simulink model "sim_v1_PD_single_coil"  (R2021b)
settings: Solver=VariableStepAuto  StartTime=0.0  StopTime=10.0  RelTol=1e-3
undefined symbols (not defined in the file or in its folder): kv, L, m, R
libraries: slpidlib x1
settings Model: Creator=User  LastModifiedBy=User

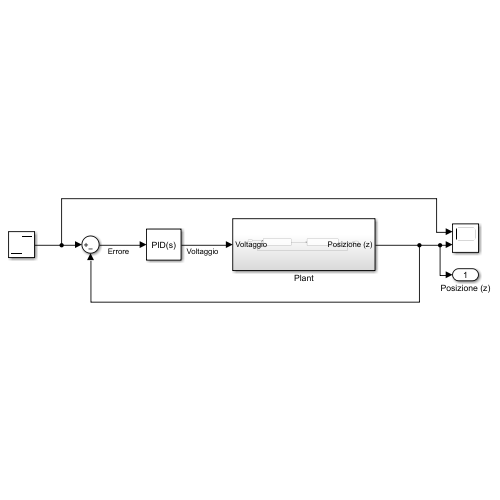
[thumbnail: Simulink's stored preview of the top-level diagram]
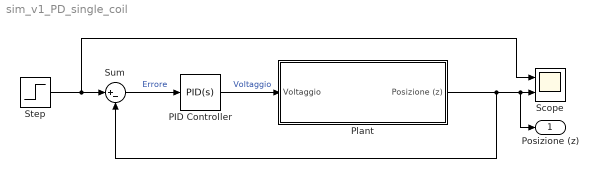
== system sim_v1_PD_single_coil ==
  PID Controller : slpidlib/PID Controller  Controller=PID  Form=Parallel  TimeDomain=Continuous-time  UseExternalTs=off  SampleTime=-1  IntegratorMethod=Forward Euler  FilterMethod=Forward Euler  ControllerParametersSource=internal  P=-1  I=1  D=1  UseFilter=on  N=100  TunerSelectOption=Transfer Function Based (PID Tuner App)  InitialConditionSource=internal  InitialConditionForIntegrator=0  InitialConditionForFilter=0  DifferentiatorICPrevScaledInput=0  ExternalReset=none  TrackingMode=off  Kt=1  LimitOutput=off  SatLimitsSource=internal  UpperSaturationLimit=inf  LowerSaturationLimit=-inf  LinearizeAsGain=on  AntiWindupMode=none  Kb=1  POutMin=[]  POutMax=[]  IOutMin=[]  IOutMax=[]  DOutMin=[]  DOutMax=[]  NOutMin=[]  NOutMax=[]  SumOutMin=[]  SumOutMax=[]  SaturationOutMin=[]  SaturationOutMax=[]  PParamMin=[]  PParamMax=[]  IParamMin=[]  IParamMax=[]  DParamMin=[]  DParamMax=[]  NParamMin=[]  NParamMax=[]  KbParamMin=[]  KbParamMax=[]  KtParamMin=[]  KtParamMax=[]  KbOutMin=[]  KbOutMax=[]  KtOutMin=[]  KtOutMax=[]  IntegratorOutMin=[]  IntegratorOutMax=[]  FilterOutMin=[]  FilterOutMax=[]  SumI1OutMin=[]  SumI1OutMax=[]  SumI2OutMin=[]  SumI2OutMax=[]  SumI3OutMin=[]  SumI3OutMax=[]  SumI4OutMin=[]  SumI4OutMax=[]  SumDOutMin=[]  SumDOutMax=[]  DifferentiatorOutMin=[]  DifferentiatorOutMax=[]  FilterDiffOutCoefMin=[]  FilterDiffOutCoefMax=[]  ReciprocalOutMin=[]  ReciprocalOutMax=[]  SumDenOutMin=[]  SumDenOutMax=[]  SumNumOutMin=[]  SumNumOutMax=[]  DivideOutMin=[]  DivideOutMax=[]  UdiffTsProdOutMin=[]  UdiffTsProdOutMax=[]  NTsProdOutMin=[]  NTsProdOutMax=[]  UintegralTsProdOutMin=[]  UintegralTsProdOutMax=[]  UngainTsProdOutMin=[]  UngainTsProdOutMax=[]  IntegratorContinuousStateAttributes=''  IntegratorStateMustResolveToSignalObject=off  IntegratorRTWStateStorageClass=Auto  FilterContinuousStateAttributes=''  FilterStateMustResolveToSignalObject=off  FilterRTWStateStorageClass=Auto  ParallelPVariant=InternalParameters  IdealPVariant=Disabled  IVariant=InternalParameters  DVariant=InternalParameters  IntegratorVariant=Continuous  SatVariant=Disabled  AWVariant=Passthrough  PCopyVariant=Disabled  TRVariant=Disabled  FdbkBlocksVariant=Forward  IdealPFdbkVariant=Disabled  SatFdbkVariant=Disabled  DerivativeFilterVariant=ContFilter  NVariant=InternalParameters  NCopyVariant=Disabled  FilterICVariant=InternalICsFilter  IntegratorICVariant=InternalICs  ExternalResetVariant=Disabled  TRSumVariant=Passthrough  SumFdbkVariant=Disabled  SumVariant=Sum_PID  TsampFilterVariant=InternalTs  TsampNgainVariant=Passthrough  TsampIntegralVariant=Passthrough  ExternalSaturationOutDataTypeStr=Inherit: Same as second input
  Plant : Subsystem
  Scope : Scope  NumInputPorts=2
  Step : Step  SampleTime=0
  Sum : Sum  Inputs=|+-
  Posizione (z) : Outport
  wires:
  Step/1 -> Scope/1, Sum/1
  Sum/1 -> PID Controller/1  "Errore"
  Plant/1(Posizione (z)) -> Sum/2, Posizione (z)/1, Scope/2
  PID Controller/1 -> Plant/1(Voltaggio)  "Voltaggio"

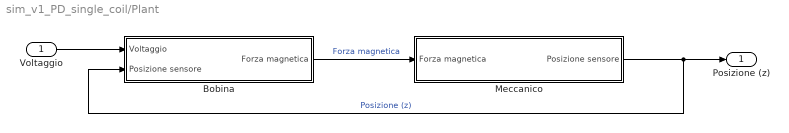
== system sim_v1_PD_single_coil/Plant ==
  Voltaggio : Inport
  Bobina : Subsystem
  Meccanico : Subsystem
  Posizione (z) : Outport
  wires:
  Bobina/1(Forza magnetica) -> Meccanico/1(Forza magnetica)  "Forza magnetica"
  Meccanico/1(Posizione sensore) -> Bobina/2(Posizione sensore), Posizione (z)/1  "Posizione (z)"
  Voltaggio/1 -> Bobina/1(Voltaggio)

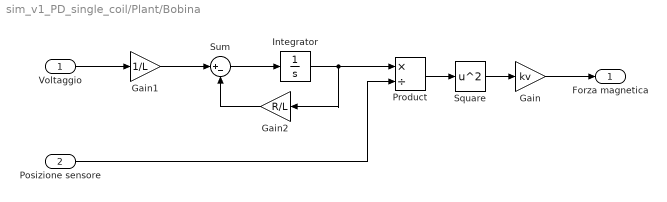
== system sim_v1_PD_single_coil/Plant/Bobina ==
  Voltaggio : Inport
  Posizione sensore : Inport  Port=2
  Gain : Gain  Gain=kv
  Gain1 : Gain  Gain=1/L
  Gain2 : Gain  Gain=R/L
  Integrator : Integrator
  Product : Product  Inputs=*/
  Square : Math  Operator=square  SaturateOnIntegerOverflow=on
  Sum : Sum  Inputs=|+-
  Forza magnetica : Outport
  wires:
  Gain/1 -> Forza magnetica/1
  Posizione sensore/1 -> Product/2
  Square/1 -> Gain/1
  Product/1 -> Square/1
  Integrator/1 -> Product/1, Gain2/1
  Voltaggio/1 -> Gain1/1
  Gain1/1 -> Sum/1
  Gain2/1 -> Sum/2
  Sum/1 -> Integrator/1

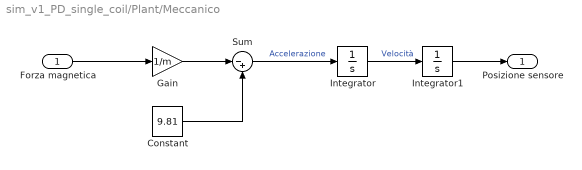
== system sim_v1_PD_single_coil/Plant/Meccanico ==
  Forza magnetica : Inport
  Constant : Constant  Value=9.81
  Gain : Gain  Gain=1/m
  Integrator : Integrator
  Integrator1 : Integrator  InitialCondition=0.02
  Sum : Sum  Inputs=|-+
  Posizione sensore : Outport
  wires:
  Forza magnetica/1 -> Gain/1
  Gain/1 -> Sum/1
  Constant/1 -> Sum/2
  Sum/1 -> Integrator/1  "Accelerazione"
  Integrator/1 -> Integrator1/1  "Velocità"
  Integrator1/1 -> Posizione sensore/1
